simulink model "control_tanque_modelo_noLineal"  (Simulink 9.2)
settings: Solver=ode4  StartTime=0.0  StopTime=700  FixedStep=0.1  RelTol=1e-3  EnableMultiTasking=on
values from neighbouring files (symbols this model uses):
  g = 9.8    [tank_parameters.m]
  Km = 2.7e-6    (= 2.7e-06)    [tank_parameters.m]
  R = 0.0295    [tank_parameters.m]
  r = 0.0015    [tank_parameters.m]
undefined symbols (not defined in the file or in its folder): magnitude, Newton, Raphson
libraries: simulink x1
settings Model: Creator=HV  LastModifiedBy=HVO
settings OptimizationCC: ExpressionDepthLimit=2147483647
settings DebuggingCC: SolverPrmCheckMsg=warning
settings ConfigComp: CovSFcnEnable=off

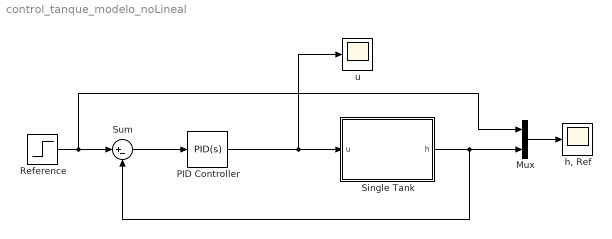
== system control_tanque_modelo_noLineal ==
  Mux : Mux  Inputs=2
  PID Controller : simulink/Continuous/PID Controller  Controller=PID  Form=Ideal  TimeDomain=Continuous-time  SampleTime=-1  IntegratorMethod=Forward Euler  FilterMethod=Forward Euler  ControllerParametersSource=internal  P=659.57  I=0.825  D=0  UseFilter=on  N=1  TunerSelectOption=Transfer Function Based (PID Tuner App)  InitialConditionSource=internal  InitialConditionForIntegrator=0  InitialConditionForFilter=0  DifferentiatorICPrevScaledInput=0  ExternalReset=none  TrackingMode=off  Kt=10  LimitOutput=off  UpperSaturationLimit=10  LowerSaturationLimit=0  LinearizeAsGain=off  AntiWindupMode=back-calculation  Kb=0.01  POutMin=[]  POutMax=[]  IOutMin=[]  IOutMax=[]  DOutMin=[]  DOutMax=[]  NOutMin=[]  NOutMax=[]  SumOutMin=[]  SumOutMax=[]  SaturationOutMin=[]  SaturationOutMax=[]  PParamMin=[]  PParamMax=[]  IParamMin=[]  IParamMax=[]  DParamMin=[]  DParamMax=[]  NParamMin=[]  NParamMax=[]  KbParamMin=[]  KbParamMax=[]  KtParamMin=[]  KtParamMax=[]  KbOutMin=[]  KbOutMax=[]  KtOutMin=[]  KtOutMax=[]  IntegratorOutMin=[]  IntegratorOutMax=[]  FilterOutMin=[]  FilterOutMax=[]  SumI1OutMin=[]  SumI1OutMax=[]  SumI2OutMin=[]  SumI2OutMax=[]  SumI3OutMin=[]  SumI3OutMax=[]  SumI4OutMin=[]  SumI4OutMax=[]  SumDOutMin=[]  SumDOutMax=[]  DifferentiatorOutMin=[]  DifferentiatorOutMax=[]  FilterDiffOutCoefMin=[]  FilterDiffOutCoefMax=[]  ReciprocalOutMin=[]  ReciprocalOutMax=[]  SumDenOutMin=[]  SumDenOutMax=[]  SumNumOutMin=[]  SumNumOutMax=[]  DivideOutMin=[]  DivideOutMax=[]  IntegratorContinuousStateAttributes=''  IntegratorStateMustResolveToSignalObject=off  IntegratorRTWStateStorageClass=Auto  FilterContinuousStateAttributes=''  FilterStateMustResolveToSignalObject=off  FilterRTWStateStorageClass=Auto  ParallelPVariant=Passthrough  IdealPVariant=InternalParameters  IVariant=InternalParameters  DVariant=InternalParameters  IntegratorVariant=Continuous  SatVariant=Disabled  AWVariant=Passthrough  PCopyVariant=Disabled  TRVariant=Disabled  FdbkBlocksVariant=Forward  IdealPFdbkVariant=Disabled  SatFdbkVariant=Disabled  DerivativeFilterVariant=ContFilter  NVariant=InternalParameters  NCopyVariant=Disabled  FilterICVariant=InternalICsFilter  IntegratorICVariant=InternalICs  ExternalResetVariant=Disabled  TRSumVariant=Passthrough  SumFdbkVariant=Disabled  SumVariant=Sum_PID
  Reference : Step  Time=500  Before=0.12  After=0.15  SampleTime=0.1
  Single Tank : Subsystem
  Sum : Sum  Inputs=|+-
  "h, Ref" : Scope
  u : Scope
  wires:
  Sum/1 -> PID Controller/1
  Single Tank/1(h) -> Mux/2, Sum/2
  Mux/1 -> "h, Ref"/1
  Reference/1 -> Mux/1, Sum/1
  PID Controller/1 -> u/1, Single Tank/1(u)

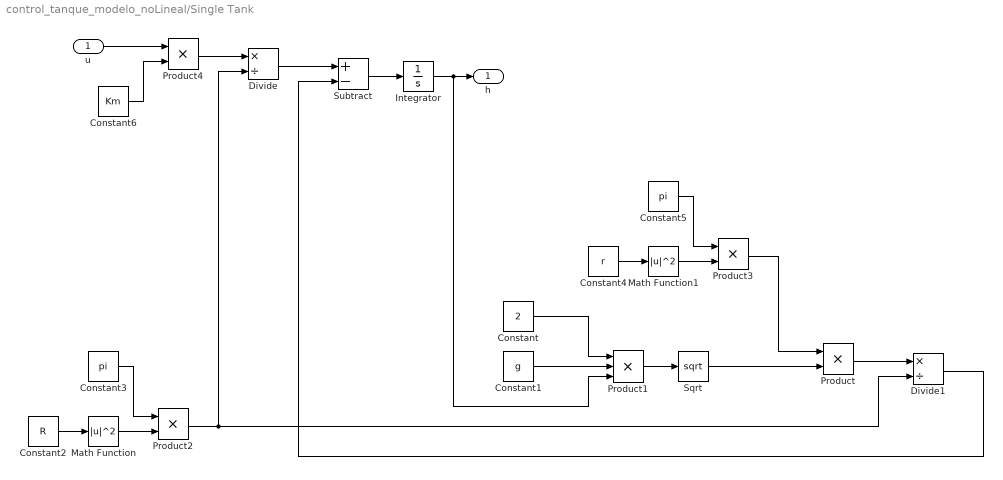
== system control_tanque_modelo_noLineal/Single Tank ==
  u : Inport
  Constant : Constant  Value=2
  Constant1 : Constant  Value=g
  Constant2 : Constant  Value=R
  Constant3 : Constant  Value=pi
  Constant4 : Constant  Value=r
  Constant5 : Constant  Value=pi
  Constant6 : Constant  Value=Km
  Divide : Product  Inputs=*/
  Divide1 : Product  Inputs=*/
  Integrator : Integrator  LimitOutput=on  LowerSaturationLimit=0
  Math Function : Math  Operator=magnitude^2  SaturateOnIntegerOverflow=on
  Math Function1 : Math  Operator=magnitude^2  SaturateOnIntegerOverflow=on
  Product{,2..4} (4 alike) : Product  RndMeth=Zero
  Product1 : Product  Inputs=3  RndMeth=Zero
  Sqrt : Sqrt  AlgorithmType=Newton-Raphson  SaturateOnIntegerOverflow=on
  Subtract : Sum  Inputs=+-
  h : Outport
  wires:
  Divide1/1 -> Subtract/2
  Product2/1 -> Divide1/2, Divide/2
  Product3/1 -> Product/1
  Constant5/1 -> Product3/1
  Constant4/1 -> Math Function1/1
  Math Function1/1 -> Product3/2
  Constant3/1 -> Product2/1
  Constant2/1 -> Math Function/1
  Math Function/1 -> Product2/2
  Product/1 -> Divide1/1
  Constant1/1 -> Product1/2
  Constant/1 -> Product1/1
  Product1/1 -> Sqrt/1
  Sqrt/1 -> Product/2
  Integrator/1 -> Product1/3, h/1
  Subtract/1 -> Integrator/1
  Divide/1 -> Subtract/1
  Product4/1 -> Divide/1
  u/1 -> Product4/1
  Constant6/1 -> Product4/2
